simulink model "TST_AFS_DD"  (R2016b)
settings: Solver=FixedStepDiscrete  StartTime=0.0  StopTime=simTime  FixedStep=sampleTime  RelTol=1e-3
values from neighbouring files (symbols this model uses):
  testCase = 1    [initTST_AFS_DD_001.m]    (also in initTST_AFS_DD_002.m = 2)
libraries: simulink x9, UnitTest_Lib x6
settings Model: Creator=zhoutinglin  LastModifiedBy=zhengjinyan
settings DebuggingCC: SignalRangeChecking=error

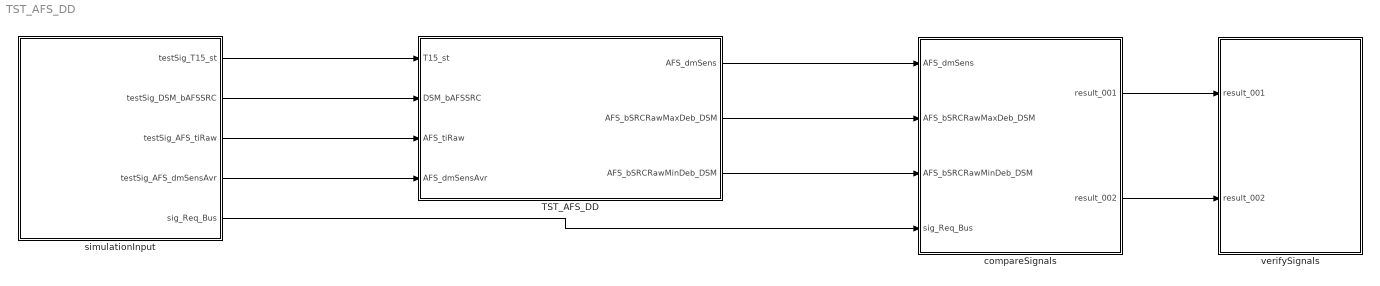
== system TST_AFS_DD ==
  TST_AFS_DD : Subsystem
  compareSignals : Subsystem
  simulationInput : Subsystem
  verifySignals : Subsystem
  wires:
  simulationInput/1(testSig_T15_st) -> TST_AFS_DD/1(T15_st)
  simulationInput/2(testSig_DSM_bAFSSRC) -> TST_AFS_DD/2(DSM_bAFSSRC)
  simulationInput/3(testSig_AFS_tiRaw) -> TST_AFS_DD/3(AFS_tiRaw)
  simulationInput/4(testSig_AFS_dmSensAvr) -> TST_AFS_DD/4(AFS_dmSensAvr)
  TST_AFS_DD/1(AFS_dmSens) -> compareSignals/1(AFS_dmSens)
  TST_AFS_DD/2(AFS_bSRCRawMaxDeb_DSM) -> compareSignals/2(AFS_bSRCRawMaxDeb_DSM)
  TST_AFS_DD/3(AFS_bSRCRawMinDeb_DSM) -> compareSignals/3(AFS_bSRCRawMinDeb_DSM)
  simulationInput/5(sig_Req_Bus) -> compareSignals/4(sig_Req_Bus)
  compareSignals/1(result_001) -> verifySignals/1(result_001)
  compareSignals/2(result_002) -> verifySignals/2(result_002)

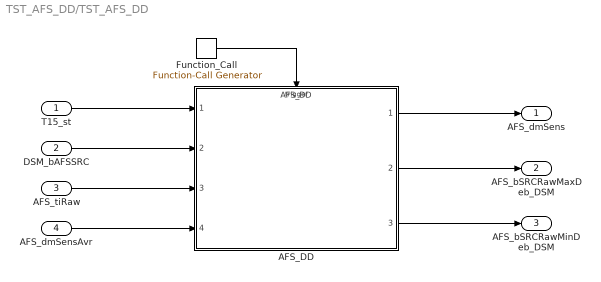
== system TST_AFS_DD/TST_AFS_DD ==
  T15_st : Inport
  DSM_bAFSSRC : Inport  Port=2
  AFS_tiRaw : Inport  Port=3
  AFS_dmSensAvr : Inport  Port=4
  AFS_DD : ModelReference  ModelNameDialog=AFS_DD  SimulationMode=Normal  ModelReferenceVersion=1.64  TriggerPortName=function  TriggerPortTriggerType=function-call  TriggerPortStatesWhenEnabling=held
  Function_Call : simulink/Ports & Subsystems/Function-Call Generator  sample_time=sampleTime  numberOfIterations=1
  AFS_dmSens : Outport
  AFS_bSRCRawMaxDeb_DSM : Outport  Port=2
  AFS_bSRCRawMinDeb_DSM : Outport  Port=3
  wires:
  Function_Call/1 -> AFS_DD/Trigger
  T15_st/1 -> AFS_DD/1
  DSM_bAFSSRC/1 -> AFS_DD/2
  AFS_tiRaw/1 -> AFS_DD/3
  AFS_dmSensAvr/1 -> AFS_DD/4
  AFS_DD/1 -> AFS_dmSens/1
  AFS_DD/2 -> AFS_bSRCRawMaxDeb_DSM/1
  AFS_DD/3 -> AFS_bSRCRawMinDeb_DSM/1

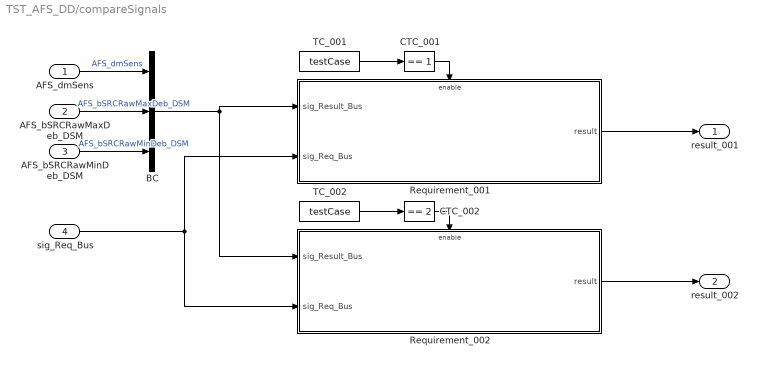
== system TST_AFS_DD/compareSignals ==
  AFS_dmSens : Inport
  AFS_bSRCRawMaxDeb_DSM : Inport  Port=2
  AFS_bSRCRawMinDeb_DSM : Inport  Port=3
  sig_Req_Bus : Inport  Port=4
  BC : BusCreator  Inputs=3
  CTC_001 : simulink/Logic and Bit Operations/Compare To Constant  relop===  const=1  OutDataTypeStr=boolean
  CTC_002 : simulink/Logic and Bit Operations/Compare To Constant  relop===  const=2  OutDataTypeStr=boolean
  Requirement_001 : Subsystem
  Requirement_002 : Subsystem
  TC_001 : Constant  Value=testCase
  TC_002 : Constant  Value=testCase
  result_001 : Outport
  result_002 : Outport  Port=2
  wires:
  AFS_dmSens/1 -> BC/1  "AFS_dmSens"
  AFS_bSRCRawMaxDeb_DSM/1 -> BC/2  "AFS_bSRCRawMaxDeb_DSM"
  AFS_bSRCRawMinDeb_DSM/1 -> BC/3  "AFS_bSRCRawMinDeb_DSM"
  TC_001/1 -> CTC_001/1
  CTC_001/1 -> Requirement_001/Enable
  sig_Req_Bus/1 -> Requirement_001/2(sig_Req_Bus), Requirement_002/2(sig_Req_Bus)
  BC/1 -> Requirement_001/1(sig_Result_Bus), Requirement_002/1(sig_Result_Bus)
  Requirement_001/1(result) -> result_001/1
  TC_002/1 -> CTC_002/1
  CTC_002/1 -> Requirement_002/Enable
  Requirement_002/1(result) -> result_002/1

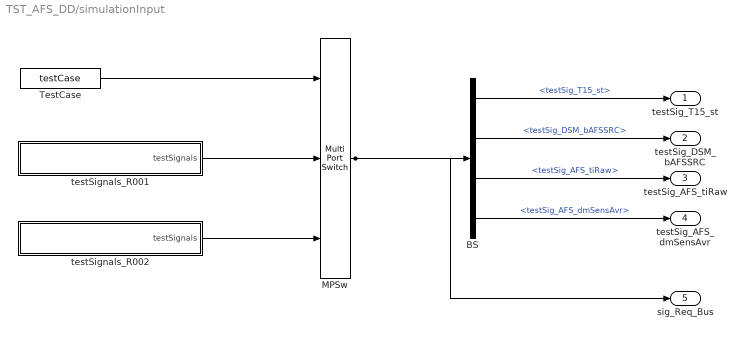
== system TST_AFS_DD/simulationInput ==
  BS : BusSelector  OutputSignals=testSig_T15_st,testSig_DSM_bAFSSRC,testSig_AFS_tiRaw,testSig_AFS_dmSensAvr
  MPSw : MultiPortSwitch  Inputs=2  SaturateOnIntegerOverflow=on  InputSameDT=on
  TestCase : Constant  Value=testCase
  testSignals_R001 : Subsystem
  testSignals_R002 : Subsystem
  testSig_T15_st : Outport
  testSig_DSM_bAFSSRC : Outport  Port=2
  testSig_AFS_tiRaw : Outport  Port=3
  testSig_AFS_dmSensAvr : Outport  Port=4
  sig_Req_Bus : Outport  Port=5
  wires:
  BS/1 -> testSig_T15_st/1  "<testSig_T15_st>"
  BS/2 -> testSig_DSM_bAFSSRC/1  "<testSig_DSM_bAFSSRC>"
  BS/3 -> testSig_AFS_tiRaw/1  "<testSig_AFS_tiRaw>"
  BS/4 -> testSig_AFS_dmSensAvr/1  "<testSig_AFS_dmSensAvr>"
  MPSw/1 -> BS/1, sig_Req_Bus/1
  TestCase/1 -> MPSw/1
  testSignals_R001/1(testSignals) -> MPSw/2
  testSignals_R002/1(testSignals) -> MPSw/3

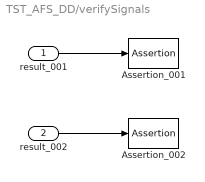
== system TST_AFS_DD/verifySignals ==
  result_001 : Inport
  result_002 : Inport  Port=2
  Assertion_001 : Assertion  Enabled=off
  Assertion_002 : Assertion  Enabled=off
  wires:
  result_001/1 -> Assertion_001/1
  result_002/1 -> Assertion_002/1

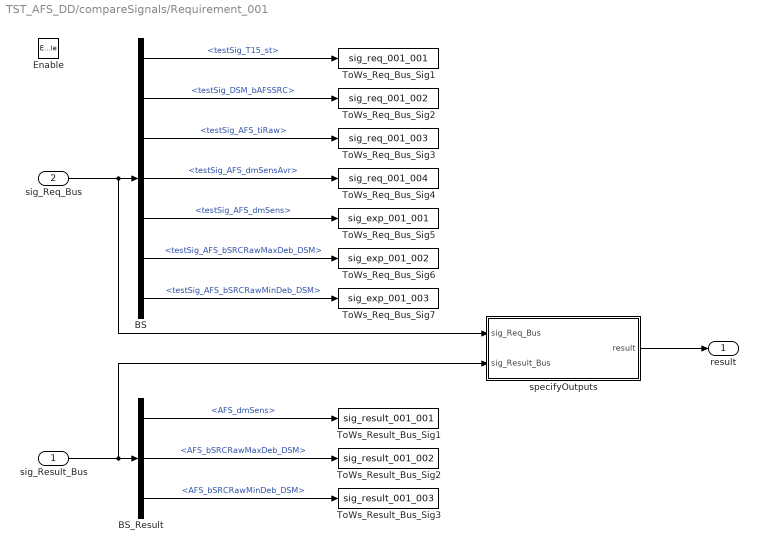
== system TST_AFS_DD/compareSignals/Requirement_001 ==
  sig_Result_Bus : Inport
  sig_Req_Bus : Inport  Port=2
  Enable : EnablePort
  BS : BusSelector  OutputSignals=testSig_T15_st,testSig_DSM_bAFSSRC,testSig_AFS_tiRaw,testSig_AFS_dmSensAvr,testSig_AFS_dmSens,testSig_AFS_bSRCRawMaxDeb_DSM,testSig_AFS_bSRCRawMinDeb_DSM
  BS_Result : BusSelector  OutputSignals=AFS_dmSens,AFS_bSRCRawMaxDeb_DSM,AFS_bSRCRawMinDeb_DSM
  ToWs_Req_Bus_Sig1 : ToWorkspace  VariableName=sig_req_001_001  SaveFormat=Structure With Time
  ToWs_Req_Bus_Sig2 : ToWorkspace  VariableName=sig_req_001_002  SaveFormat=Structure With Time
  ToWs_Req_Bus_Sig3 : ToWorkspace  VariableName=sig_req_001_003  SaveFormat=Structure With Time
  ToWs_Req_Bus_Sig4 : ToWorkspace  VariableName=sig_req_001_004  SaveFormat=Structure With Time
  ToWs_Req_Bus_Sig5 : ToWorkspace  VariableName=sig_exp_001_001  SaveFormat=Structure With Time
  ToWs_Req_Bus_Sig6 : ToWorkspace  VariableName=sig_exp_001_002  SaveFormat=Structure With Time
  ToWs_Req_Bus_Sig7 : ToWorkspace  VariableName=sig_exp_001_003  SaveFormat=Structure With Time
  ToWs_Result_Bus_Sig1 : ToWorkspace  VariableName=sig_result_001_001  SaveFormat=Structure With Time
  ToWs_Result_Bus_Sig2 : ToWorkspace  VariableName=sig_result_001_002  SaveFormat=Structure With Time
  ToWs_Result_Bus_Sig3 : ToWorkspace  VariableName=sig_result_001_003  SaveFormat=Structure With Time
  specifyOutputs : Subsystem
  result : Outport
  wires:
  sig_Req_Bus/1 -> BS/1, specifyOutputs/1(sig_Req_Bus)
  BS/1 -> ToWs_Req_Bus_Sig1/1  "<testSig_T15_st>"
  BS/2 -> ToWs_Req_Bus_Sig2/1  "<testSig_DSM_bAFSSRC>"
  BS/3 -> ToWs_Req_Bus_Sig3/1  "<testSig_AFS_tiRaw>"
  BS/4 -> ToWs_Req_Bus_Sig4/1  "<testSig_AFS_dmSensAvr>"
  BS/5 -> ToWs_Req_Bus_Sig5/1  "<testSig_AFS_dmSens>"
  BS/6 -> ToWs_Req_Bus_Sig6/1  "<testSig_AFS_bSRCRawMaxDeb_DSM>"
  BS/7 -> ToWs_Req_Bus_Sig7/1  "<testSig_AFS_bSRCRawMinDeb_DSM>"
  sig_Result_Bus/1 -> BS_Result/1, specifyOutputs/2(sig_Result_Bus)
  BS_Result/1 -> ToWs_Result_Bus_Sig1/1  "<AFS_dmSens>"
  BS_Result/2 -> ToWs_Result_Bus_Sig2/1  "<AFS_bSRCRawMaxDeb_DSM>"
  BS_Result/3 -> ToWs_Result_Bus_Sig3/1  "<AFS_bSRCRawMinDeb_DSM>"
  specifyOutputs/1(result) -> result/1

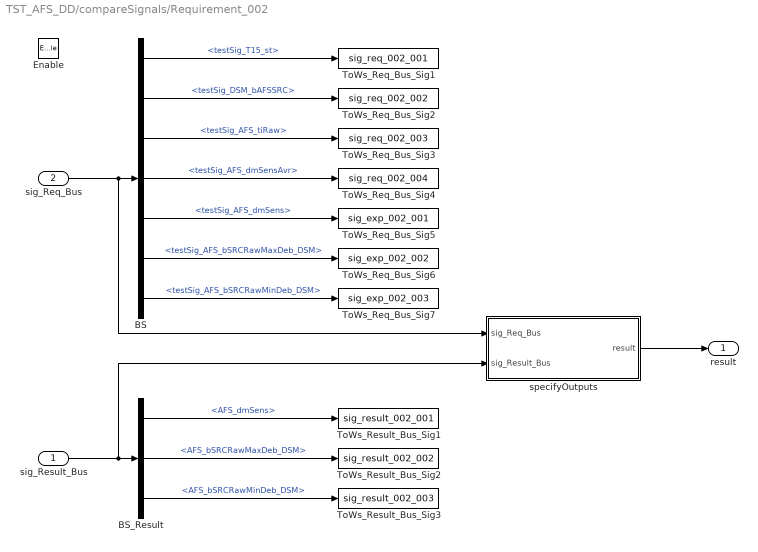
== system TST_AFS_DD/compareSignals/Requirement_002 ==
  sig_Result_Bus : Inport
  sig_Req_Bus : Inport  Port=2
  Enable : EnablePort
  BS : BusSelector  OutputSignals=testSig_T15_st,testSig_DSM_bAFSSRC,testSig_AFS_tiRaw,testSig_AFS_dmSensAvr,testSig_AFS_dmSens,testSig_AFS_bSRCRawMaxDeb_DSM,testSig_AFS_bSRCRawMinDeb_DSM
  BS_Result : BusSelector  OutputSignals=AFS_dmSens,AFS_bSRCRawMaxDeb_DSM,AFS_bSRCRawMinDeb_DSM
  ToWs_Req_Bus_Sig1 : ToWorkspace  VariableName=sig_req_002_001  SaveFormat=Structure With Time
  ToWs_Req_Bus_Sig2 : ToWorkspace  VariableName=sig_req_002_002  SaveFormat=Structure With Time
  ToWs_Req_Bus_Sig3 : ToWorkspace  VariableName=sig_req_002_003  SaveFormat=Structure With Time
  ToWs_Req_Bus_Sig4 : ToWorkspace  VariableName=sig_req_002_004  SaveFormat=Structure With Time
  ToWs_Req_Bus_Sig5 : ToWorkspace  VariableName=sig_exp_002_001  SaveFormat=Structure With Time
  ToWs_Req_Bus_Sig6 : ToWorkspace  VariableName=sig_exp_002_002  SaveFormat=Structure With Time
  ToWs_Req_Bus_Sig7 : ToWorkspace  VariableName=sig_exp_002_003  SaveFormat=Structure With Time
  ToWs_Result_Bus_Sig1 : ToWorkspace  VariableName=sig_result_002_001  SaveFormat=Structure With Time
  ToWs_Result_Bus_Sig2 : ToWorkspace  VariableName=sig_result_002_002  SaveFormat=Structure With Time
  ToWs_Result_Bus_Sig3 : ToWorkspace  VariableName=sig_result_002_003  SaveFormat=Structure With Time
  specifyOutputs : Subsystem
  result : Outport
  wires:
  sig_Req_Bus/1 -> BS/1, specifyOutputs/1(sig_Req_Bus)
  BS/1 -> ToWs_Req_Bus_Sig1/1  "<testSig_T15_st>"
  BS/2 -> ToWs_Req_Bus_Sig2/1  "<testSig_DSM_bAFSSRC>"
  BS/3 -> ToWs_Req_Bus_Sig3/1  "<testSig_AFS_tiRaw>"
  BS/4 -> ToWs_Req_Bus_Sig4/1  "<testSig_AFS_dmSensAvr>"
  BS/5 -> ToWs_Req_Bus_Sig5/1  "<testSig_AFS_dmSens>"
  BS/6 -> ToWs_Req_Bus_Sig6/1  "<testSig_AFS_bSRCRawMaxDeb_DSM>"
  BS/7 -> ToWs_Req_Bus_Sig7/1  "<testSig_AFS_bSRCRawMinDeb_DSM>"
  sig_Result_Bus/1 -> BS_Result/1, specifyOutputs/2(sig_Result_Bus)
  BS_Result/1 -> ToWs_Result_Bus_Sig1/1  "<AFS_dmSens>"
  BS_Result/2 -> ToWs_Result_Bus_Sig2/1  "<AFS_bSRCRawMaxDeb_DSM>"
  BS_Result/3 -> ToWs_Result_Bus_Sig3/1  "<AFS_bSRCRawMinDeb_DSM>"
  specifyOutputs/1(result) -> result/1

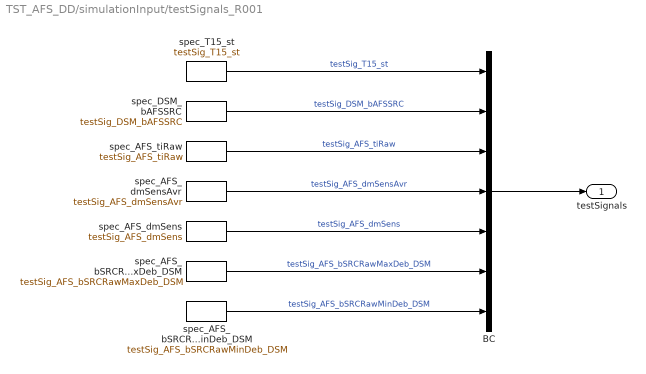
== system TST_AFS_DD/simulationInput/testSignals_R001 ==
  BC : BusCreator  Inputs=7
  spec_AFS_bSRCRawMaxDeb_DSM : FromWorkspace  VariableName=testSig_AFS_bSRCRawMaxDeb_DSM  Interpolate=off  OutputAfterFinalValue=Holding final value
  spec_AFS_bSRCRawMinDeb_DSM : FromWorkspace  VariableName=testSig_AFS_bSRCRawMinDeb_DSM  Interpolate=off  OutputAfterFinalValue=Holding final value
  spec_AFS_dmSens : FromWorkspace  VariableName=testSig_AFS_dmSens  Interpolate=off  OutputAfterFinalValue=Holding final value
  spec_AFS_dmSensAvr : FromWorkspace  VariableName=testSig_AFS_dmSensAvr  Interpolate=off  OutputAfterFinalValue=Holding final value
  spec_AFS_tiRaw : FromWorkspace  VariableName=testSig_AFS_tiRaw  Interpolate=off  OutputAfterFinalValue=Holding final value
  spec_DSM_bAFSSRC : FromWorkspace  VariableName=testSig_DSM_bAFSSRC  Interpolate=off  OutputAfterFinalValue=Holding final value
  spec_T15_st : FromWorkspace  VariableName=testSig_T15_st  Interpolate=off  OutputAfterFinalValue=Holding final value
  testSignals : Outport
  wires:
  BC/1 -> testSignals/1
  spec_T15_st/1 -> BC/1  "testSig_T15_st"
  spec_DSM_bAFSSRC/1 -> BC/2  "testSig_DSM_bAFSSRC"
  spec_AFS_tiRaw/1 -> BC/3  "testSig_AFS_tiRaw"
  spec_AFS_dmSensAvr/1 -> BC/4  "testSig_AFS_dmSensAvr"
  spec_AFS_dmSens/1 -> BC/5  "testSig_AFS_dmSens"
  spec_AFS_bSRCRawMaxDeb_DSM/1 -> BC/6  "testSig_AFS_bSRCRawMaxDeb_DSM"
  spec_AFS_bSRCRawMinDeb_DSM/1 -> BC/7  "testSig_AFS_bSRCRawMinDeb_DSM"

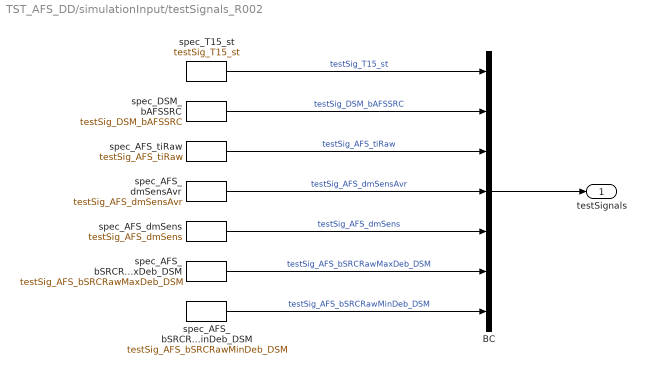
== system TST_AFS_DD/simulationInput/testSignals_R002 ==
  BC : BusCreator  Inputs=7
  spec_AFS_bSRCRawMaxDeb_DSM : FromWorkspace  VariableName=testSig_AFS_bSRCRawMaxDeb_DSM  Interpolate=off  OutputAfterFinalValue=Holding final value
  spec_AFS_bSRCRawMinDeb_DSM : FromWorkspace  VariableName=testSig_AFS_bSRCRawMinDeb_DSM  Interpolate=off  OutputAfterFinalValue=Holding final value
  spec_AFS_dmSens : FromWorkspace  VariableName=testSig_AFS_dmSens  Interpolate=off  OutputAfterFinalValue=Holding final value
  spec_AFS_dmSensAvr : FromWorkspace  VariableName=testSig_AFS_dmSensAvr  Interpolate=off  OutputAfterFinalValue=Holding final value
  spec_AFS_tiRaw : FromWorkspace  VariableName=testSig_AFS_tiRaw  Interpolate=off  OutputAfterFinalValue=Holding final value
  spec_DSM_bAFSSRC : FromWorkspace  VariableName=testSig_DSM_bAFSSRC  Interpolate=off  OutputAfterFinalValue=Holding final value
  spec_T15_st : FromWorkspace  VariableName=testSig_T15_st  Interpolate=off  OutputAfterFinalValue=Holding final value
  testSignals : Outport
  wires:
  BC/1 -> testSignals/1
  spec_T15_st/1 -> BC/1  "testSig_T15_st"
  spec_DSM_bAFSSRC/1 -> BC/2  "testSig_DSM_bAFSSRC"
  spec_AFS_tiRaw/1 -> BC/3  "testSig_AFS_tiRaw"
  spec_AFS_dmSensAvr/1 -> BC/4  "testSig_AFS_dmSensAvr"
  spec_AFS_dmSens/1 -> BC/5  "testSig_AFS_dmSens"
  spec_AFS_bSRCRawMaxDeb_DSM/1 -> BC/6  "testSig_AFS_bSRCRawMaxDeb_DSM"
  spec_AFS_bSRCRawMinDeb_DSM/1 -> BC/7  "testSig_AFS_bSRCRawMinDeb_DSM"

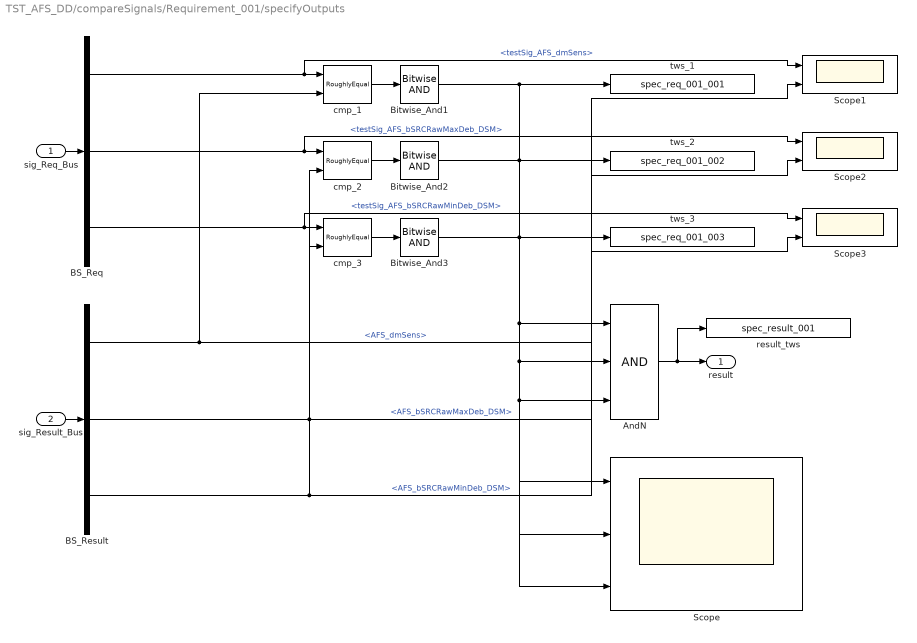
== system TST_AFS_DD/compareSignals/Requirement_001/specifyOutputs ==
  sig_Req_Bus : Inport
  sig_Result_Bus : Inport  Port=2
  AndN : Logic  Inputs=3
  BS_Req : BusSelector  OutputSignals=testSig_AFS_dmSens,testSig_AFS_bSRCRawMaxDeb_DSM,testSig_AFS_bSRCRawMinDeb_DSM
  BS_Result : BusSelector  OutputSignals=AFS_dmSens,AFS_bSRCRawMaxDeb_DSM,AFS_bSRCRawMinDeb_DSM
  Bitwise_And1 : simulink/Logic and Bit Operations/Bitwise Operator  logicop=AND  UseBitMask=off  BitMask=bin2dec('11011001')  BitMaskRealWorld=Stored Integer
  Bitwise_And2 : simulink/Logic and Bit Operations/Bitwise Operator  logicop=AND  UseBitMask=off  BitMask=bin2dec('11011001')  BitMaskRealWorld=Stored Integer
  Bitwise_And3 : simulink/Logic and Bit Operations/Bitwise Operator  logicop=AND  UseBitMask=off  BitMask=bin2dec('11011001')  BitMaskRealWorld=Stored Integer
  Scope : Scope  NumInputPorts=3
  Scope1 : Scope  NumInputPorts=2
  Scope2 : Scope  NumInputPorts=2
  Scope3 : Scope  NumInputPorts=2
  cmp_1 : UnitTest_Lib/RoughlyEqual  slope=10
  cmp_2 : UnitTest_Lib/RoughlyEqual  slope=1
  cmp_3 : UnitTest_Lib/RoughlyEqual  slope=1
  result_tws : ToWorkspace  VariableName=spec_result_001
  tws_1 : ToWorkspace  VariableName=spec_req_001_001
  tws_2 : ToWorkspace  VariableName=spec_req_001_002
  tws_3 : ToWorkspace  VariableName=spec_req_001_003
  result : Outport
  wires:
  sig_Req_Bus/1 -> BS_Req/1
  sig_Result_Bus/1 -> BS_Result/1
  AndN/1 -> result/1, result_tws/1
  BS_Req/1 -> cmp_1/1, Scope1/1  "<testSig_AFS_dmSens>"
  BS_Result/1 -> cmp_1/2, Scope1/2  "<AFS_dmSens>"
  cmp_1/1 -> Bitwise_And1/1
  Bitwise_And1/1 -> AndN/1, Scope/1, tws_1/1
  BS_Req/2 -> cmp_2/1, Scope2/1  "<testSig_AFS_bSRCRawMaxDeb_DSM>"
  BS_Result/2 -> cmp_2/2, Scope2/2  "<AFS_bSRCRawMaxDeb_DSM>"
  cmp_2/1 -> Bitwise_And2/1
  Bitwise_And2/1 -> AndN/2, Scope/2, tws_2/1
  BS_Req/3 -> cmp_3/1, Scope3/1  "<testSig_AFS_bSRCRawMinDeb_DSM>"
  BS_Result/3 -> cmp_3/2, Scope3/2  "<AFS_bSRCRawMinDeb_DSM>"
  cmp_3/1 -> Bitwise_And3/1
  Bitwise_And3/1 -> AndN/3, Scope/3, tws_3/1

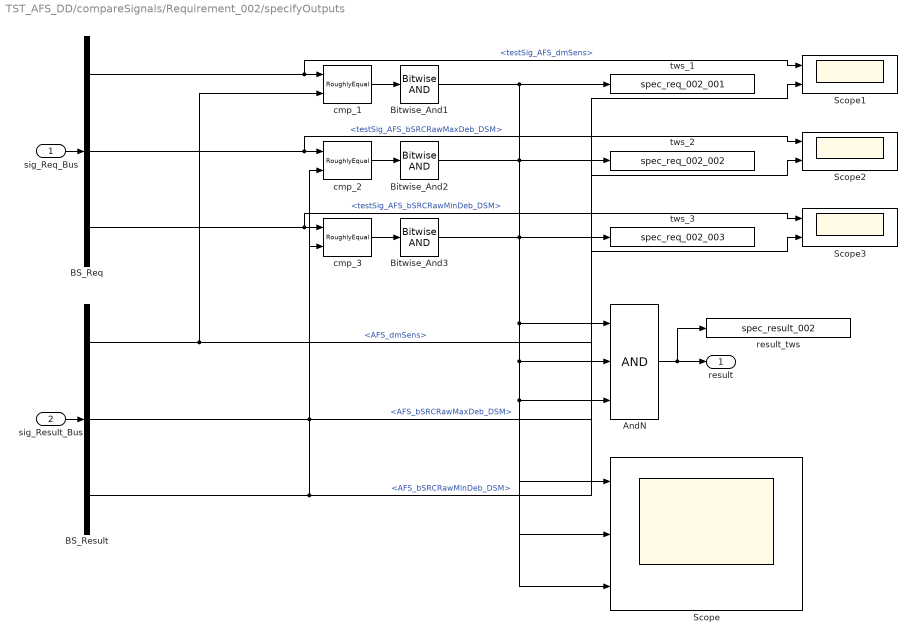
== system TST_AFS_DD/compareSignals/Requirement_002/specifyOutputs ==
  sig_Req_Bus : Inport
  sig_Result_Bus : Inport  Port=2
  AndN : Logic  Inputs=3
  BS_Req : BusSelector  OutputSignals=testSig_AFS_dmSens,testSig_AFS_bSRCRawMaxDeb_DSM,testSig_AFS_bSRCRawMinDeb_DSM
  BS_Result : BusSelector  OutputSignals=AFS_dmSens,AFS_bSRCRawMaxDeb_DSM,AFS_bSRCRawMinDeb_DSM
  Bitwise_And1 : simulink/Logic and Bit Operations/Bitwise Operator  logicop=AND  UseBitMask=off  BitMask=bin2dec('11011001')  BitMaskRealWorld=Stored Integer
  Bitwise_And2 : simulink/Logic and Bit Operations/Bitwise Operator  logicop=AND  UseBitMask=off  BitMask=bin2dec('11011001')  BitMaskRealWorld=Stored Integer
  Bitwise_And3 : simulink/Logic and Bit Operations/Bitwise Operator  logicop=AND  UseBitMask=off  BitMask=bin2dec('11011001')  BitMaskRealWorld=Stored Integer
  Scope : Scope  NumInputPorts=3
  Scope1 : Scope  NumInputPorts=2
  Scope2 : Scope  NumInputPorts=2
  Scope3 : Scope  NumInputPorts=2
  cmp_1 : UnitTest_Lib/RoughlyEqual  slope=10
  cmp_2 : UnitTest_Lib/RoughlyEqual  slope=1
  cmp_3 : UnitTest_Lib/RoughlyEqual  slope=1
  result_tws : ToWorkspace  VariableName=spec_result_002
  tws_1 : ToWorkspace  VariableName=spec_req_002_001
  tws_2 : ToWorkspace  VariableName=spec_req_002_002
  tws_3 : ToWorkspace  VariableName=spec_req_002_003
  result : Outport
  wires:
  sig_Req_Bus/1 -> BS_Req/1
  sig_Result_Bus/1 -> BS_Result/1
  AndN/1 -> result/1, result_tws/1
  BS_Req/1 -> cmp_1/1, Scope1/1  "<testSig_AFS_dmSens>"
  BS_Result/1 -> cmp_1/2, Scope1/2  "<AFS_dmSens>"
  cmp_1/1 -> Bitwise_And1/1
  Bitwise_And1/1 -> AndN/1, Scope/1, tws_1/1
  BS_Req/2 -> cmp_2/1, Scope2/1  "<testSig_AFS_bSRCRawMaxDeb_DSM>"
  BS_Result/2 -> cmp_2/2, Scope2/2  "<AFS_bSRCRawMaxDeb_DSM>"
  cmp_2/1 -> Bitwise_And2/1
  Bitwise_And2/1 -> AndN/2, Scope/2, tws_2/1
  BS_Req/3 -> cmp_3/1, Scope3/1  "<testSig_AFS_bSRCRawMinDeb_DSM>"
  BS_Result/3 -> cmp_3/2, Scope3/2  "<AFS_bSRCRawMinDeb_DSM>"
  cmp_3/1 -> Bitwise_And3/1
  Bitwise_And3/1 -> AndN/3, Scope/3, tws_3/1
